simulink model "EKFsim"  (R2025b)
settings: Solver=ode4  StartTime=0.0  StopTime=12000  FixedStep=0.01  RelTol=1e-3
values from neighbouring files (symbols this model uses):
  muE = 3.986004419e14    (= 398600441900000)    [EKF_Code.m]
  P0 = diag([10e03^2*ones(1,3), 100^2*ones(1,3), 1e-04])    [EKF_Code.m]
  Qk = diag([qPos qPos qPos qVel qVel qVel qBias])    [EKF_Code.m]
  wE = 7292115.1467e-11    (= 7.2921151467e-05)    [EKF_Code.m]    (also in ekf.m = [0;0;wE])
  x0 = [ 1.9393e6 ... (first row only)    [EKF_Code.m]
settings Model: Creator=nimis  LastModifiedBy=nimis

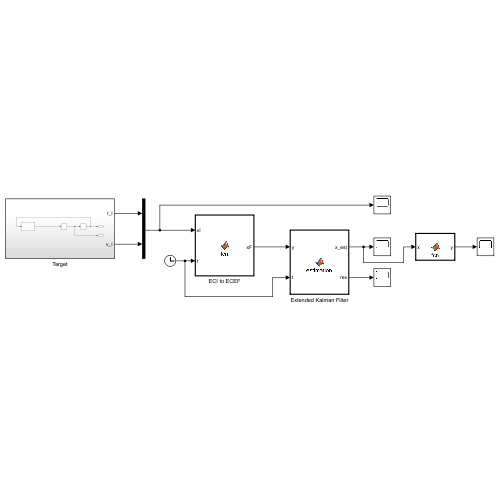
[thumbnail: Simulink's stored preview of the top-level diagram]
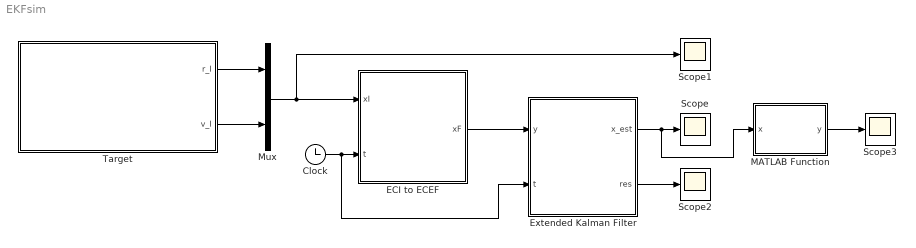
== system EKFsim ==
  Clock : Clock
  ECI to ECEF : MATLAB Function  TreatAsAtomicUnit=on
  Extended Kalman Filter : MATLAB Function  TreatAsAtomicUnit=on
  MATLAB Function : MATLAB Function  TreatAsAtomicUnit=on
  Mux : Mux  Inputs=2
  Scope{,1..3} (4 alike) : Scope
      Scope settings: ActiveDisplayYMinimum=-8.4428989798741359E+6  ActiveDisplayYMaximum=8.51678651122442E+6
      Scope1 settings: ActiveDisplayYMinimum=-8.442898612509178E+6  ActiveDisplayYMaximum=8.5167861516645681E+6
      Scope2 settings: ActiveDisplayYMinimum=-1  ActiveDisplayYMaximum=1  DataLoggingVariableName=ScopeData2
      Scope3 settings: ActiveDisplayYMinimum=362.18338150333716  ActiveDisplayYMaximum=463.68611561497141  DataLoggingVariableName=ScopeData3
  Target : Subsystem
  wires:
  Target/2(v_I) -> Mux/2
  Target/1(r_I) -> Mux/1
  Mux/1 -> Scope1/1, ECI to ECEF/1(xI)
  Clock/1 -> Extended Kalman Filter/2(t), ECI to ECEF/2(t)
  ECI to ECEF/1(xF) -> Extended Kalman Filter/1(y)
  Extended Kalman Filter/1(x_est) -> MATLAB Function/1(x), Scope/1
  Extended Kalman Filter/2(res) -> Scope2/1
  MATLAB Function/1(y) -> Scope3/1

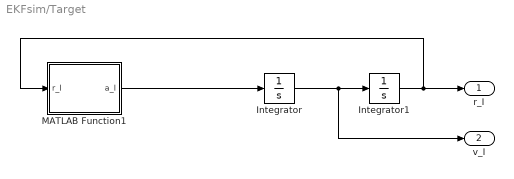
== system EKFsim/Target ==
  Integrator : Integrator  InitialCondition=x0(4:6)
  Integrator1 : Integrator  InitialCondition=x0(1:3)
  MATLAB Function1 : MATLAB Function  TreatAsAtomicUnit=on
  r_I : Outport
  v_I : Outport  Port=2
  wires:
  Integrator/1 -> v_I/1, Integrator1/1
  MATLAB Function1/1(a_I) -> Integrator/1
  Integrator1/1 -> r_I/1, MATLAB Function1/1(r_I)

== matlab function EKFsim/Extended Kalman Filter ==
  settings: updateMethod=DISCRETE  sampleTime=0.01
  data: y input; x_est output; x0 parameter; P0 parameter; muE parameter; wE parameter; Qk parameter; t input; res output
function [x_est,res] = estimation(y,x0,P0,muE,wE,Qk,t)

est   = ekf(y,x0,P0,muE,wE,Qk,t);
x_est = est.x_est;
res   = est.res;

end

== matlab function EKFsim/ECI to ECEF ==
  data: xI input; xF output; t input; wE parameter
function xF = fcn(xI, t, wE)

C_FI = rotate_z(wE*t);

wE = [0;0;wE];

xF = [C_FI*xI(1:3); -skew(wE)*C_FI*xI(1:3) + C_FI*xI(4:6)];

end

== matlab function EKFsim/MATLAB Function ==
  data: x input; y output; rEarth_km parameter
function y = fcn(x, rEarth_km)

y = norm(x)*1e-03-rEarth_km;

== matlab function EKFsim/Target/MATLAB Function1 ==
  settings: updateMethod=CONTINUOUS  sampleTime=baseRate
  data: r_I input; a_I output; muE parameter
function a_I = fcn(r_I, muE)

a_I = r_I .* (-muE / (norm(r_I)^3));

end
